simulink model "ex_3"  (R2019a)
settings: Solver=FixedStepAuto  StartTime=0.0  StopTime=inf  FixedStep=1  RelTol=1e-3
settings Model: Creator=anton  LastModifiedBy=anton

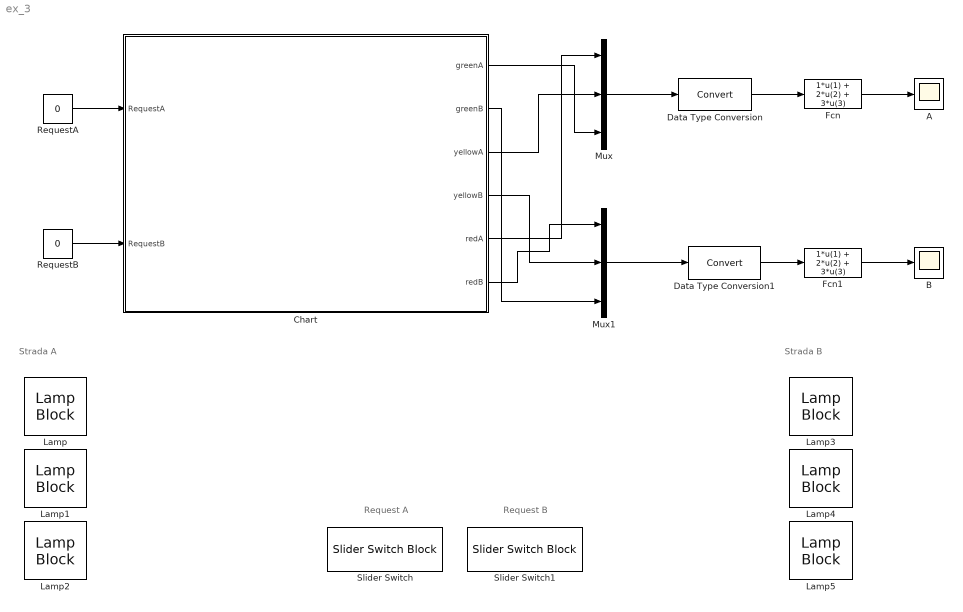
== system ex_3 ==
  note: Request A
  note: Strada A
  note: Strada B
  note: Request B
  A : Scope
  B : Scope
  Chart : Stateflow chart  BlockKeywords=__PRM__SERIALIZED__DATA__:Stateflow Chart,Stateflow Diagram  TreatAsAtomicUnit=on
  Data Type Conversion : DataTypeConversion
  Data Type Conversion1 : DataTypeConversion
  Fcn : Fcn  Expr=1*u(1) + 2*u(2) + 3*u(3)
  Fcn1 : Fcn  Expr=1*u(1) + 2*u(2) + 3*u(3)
  Lamp{,1..5} (6 alike) : LampBlock
  Mux : Mux  Inputs=3
  Mux1 : Mux  Inputs=3
  RequestA : Constant  Value=0
  RequestB : Constant  Value=0
  Slider Switch : SliderSwitchBlock
      settings: Values={{'Off', 'On'}, [0 1]}
  Slider Switch1 : SliderSwitchBlock
      settings: Values={{'Off', 'On'}, [0 1]}
  wires:
  Chart/1(greenA) -> Mux/3
  Chart/3(yellowA) -> Mux/2
  Chart/5(redA) -> Mux/1
  Chart/6(redB) -> Mux1/1
  Chart/4(yellowB) -> Mux1/2
  Chart/2(greenB) -> Mux1/3
  RequestA/1 -> Chart/1(RequestA)
  RequestB/1 -> Chart/2(RequestB)
  Fcn/1 -> A/1
  Fcn1/1 -> B/1
  Mux/1 -> Data Type Conversion/1
  Data Type Conversion/1 -> Fcn/1
  Mux1/1 -> Data Type Conversion1/1
  Data Type Conversion1/1 -> Fcn1/1

== stateflow chart ex_3/Chart ==
  state A [parallel]
    settings: executionOrder=1
    state RedA
      greenA=false;
      yellowA=false;
      redA = true;
      pause(0.4);
    state WaitForRedB
      redRequestB = true;
      pause(0.4);
    state GreenA
      redA=false;
      yellowA=false;
      greenA=true;
      redRequestB=false;
      pause(0.4);
    state YellowA
      redA=false;
      yellowA=true;
      greenA=false;
      pause(0.4);
    (default) -> RedA : {redRequestA =false;redRequestB=false}
    RedA -> WaitForRedB : [(after(40,sec)) || (after(20,sec) && RequestA == 1)]
    YellowA -> RedA : [after(5,sec)]
    WaitForRedB -> GreenA : [redB==true]
    GreenA -> YellowA : [after(35,sec) || redRequestA == true]
  state B [parallel]
    settings: executionOrder=2
    state RedB
      greenB=false;
      yellowB=false;
      redB=true;
    state WaitForRedA
      redRequestA = true;
    state GreenB
      redB=false;
      yellowB=false;
      greenB=true;
      redRequestA=false;
    state YellowB
      redB=false;
      yellowB=true;
      greenB=false;
    (default) -> RedB : {redRequestA =false;redRequestB=false}
    RedB -> WaitForRedA : [after(60,sec) || (after(40,sec) && RequestB == 1)]
    WaitForRedA -> GreenB : [redA == true]
    YellowB -> RedB : [after(5,sec)]
    GreenB -> YellowB : [after(35,sec) || redRequestB == true]
  data: greenA output; greenB output; yellowA output; yellowB output; redA output; redB output; RequestA input; RequestB input; redRequestA local; redRequestB local
